simulink model "miniproject2"  (R2015a)
settings: Solver=ode45  StartTime=0.0  StopTime=0.1  RelTol=1e-3
undefined symbols (not defined in the file): D1, Delta
libraries: powerlib x18, powerlib_meascontrol x4
settings Model: Creator=ASUS  LastModifiedBy=ASUS

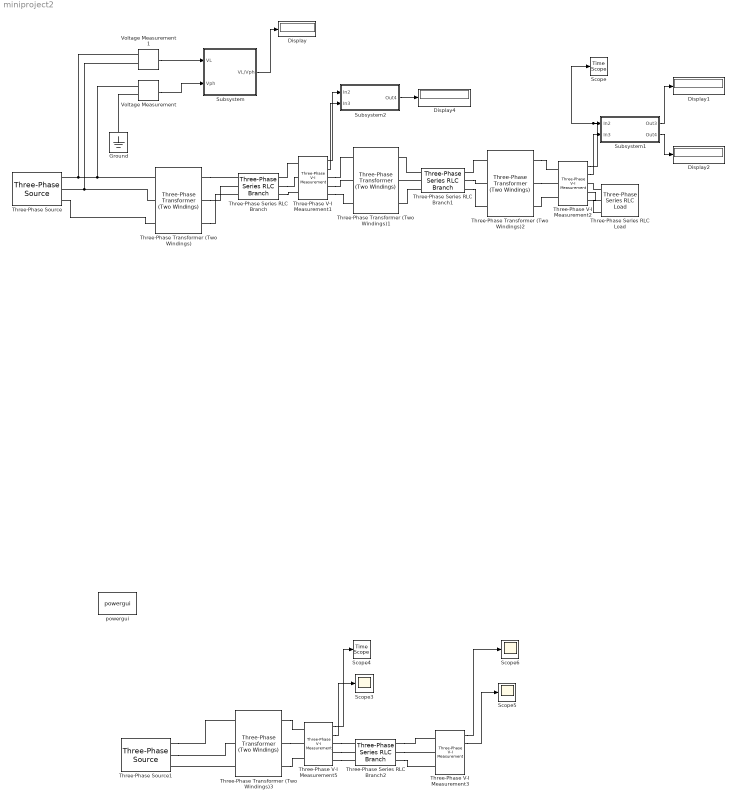
== system miniproject2 ==
  Display{,1..2,4} (4 alike) : Display
  Ground : powerlib/Elements/Ground  LConnTagsString=a
  Scope : TimeScope
  Scope3 : Scope
      settings: SaveName=ScopeData3
  Scope4 : TimeScope
  Scope5 : Scope
      settings: SaveName=ScopeData5
  Scope6 : Scope
      settings: SaveName=ScopeData8
  Subsystem : Subsystem
  Subsystem1 : Subsystem
  Subsystem2 : Subsystem
  Three-Phase Series RLC Branch : powerlib/Elements/Three-Phase Series RLC Branch  LConnTagsString=A|B|C  RConnTagsString=A|B|C  BranchType=RL  Resistance=271*0.01  Inductance=271*0.01  Capacitance=1e-6  Measurements=None
  Three-Phase Series RLC Branch1 : powerlib/Elements/Three-Phase Series RLC Branch  LConnTagsString=A|B|C  RConnTagsString=A|B|C  BranchType=RL  Resistance=(5+10^-3*171)  Inductance=(5+10^-3*171)  Capacitance=1e-6  Measurements=None
  Three-Phase Series RLC Branch2 : powerlib/Elements/Three-Phase Series RLC Branch  LConnTagsString=A|B|C  RConnTagsString=A|B|C  BranchType=RL  Resistance=271*0.01  Inductance=271*0.01  Capacitance=1e-6  Measurements=None
  Three-Phase Series RLC Load : powerlib/Elements/Three-Phase Series RLC Load  LConnTagsString=A|B|C  Configuration=Y (grounded)  NominalVoltage=1000  NominalFrequency=50  ActivePower=1000000  InductivePower=0.5e6  CapacitivePower=0  Measurements=None  LoadType=constant Z
  Three-Phase Transformer (Two Windings) : powerlib/Elements/Three-Phase Transformer (Two Windings)  Winding1Connection=Delta (D1)  Winding2Connection=Yg  CoreType=Three single-phase transformers  SetSaturation=off  Hysteresis=off  DataFile='hysteresis'  SetInitialFlux=off  Measurements=None  UNITS=pu  NominalPower=[ 250e6 , 50 ]  Winding1=[11000 0.0013774 17.309]  Winding2=[2.3e+05 9.4518e-06 0.11877]  Rm=344.35  Lm=1.0818e+05  L0=108.18  Saturation=[0 0;2.2401e-07 0.024234;9.3338e-05 0.030696]  InitialFluxes=[0.016156 -0.016156 0.014136]  MoreParameters=off  BreakLoop=off  DataType=off  TransfoNumber=1
  Three-Phase Transformer (Two Windings)1 : powerlib/Elements/Three-Phase Transformer (Two Windings)  Winding1Connection=Yg  Winding2Connection=Delta (D1)  CoreType=Three single-phase transformers  SetSaturation=off  Hysteresis=off  DataFile='hysteresis'  SetInitialFlux=off  Measurements=None  UNITS=SI  NominalPower=[ 450e6 , 50 ]  Winding1=[2.3e+05 6.5308e-07 5.8508e-13]  Winding2=[11000 2.2295e+09 1997.4]  Rm=0.16327  Lm=3.6568e-09  L0=8.2715e-07  Saturation=[0 0;6.901e+11 2523.6;2.8755e+14 3196.6]  InitialFluxes=[1682.4 -1682.4 1472.1]  MoreParameters=off  BreakLoop=off  DataType=on  TransfoNumber=1
  Three-Phase Transformer (Two Windings)2 : powerlib/Elements/Three-Phase Transformer (Two Windings)  Winding1Connection=Yg  Winding2Connection=Yg  CoreType=Three single-phase transformers  SetSaturation=off  Hysteresis=off  DataFile='hysteresis'  SetInitialFlux=off  Measurements=None  UNITS=pu  NominalPower=[ 450e6 , 50 ]  Winding1=[11000 0.007438 93.469]  Winding2=[400 5.625 70686]  Rm=1859.5  Lm=5.8418e+05  L0=584.18  Saturation=[0 0;7.1852e-08 0.041974;2.9938e-05 0.053168]  InitialFluxes=[0.027983 -0.027983 0.024485]  MoreParameters=off  BreakLoop=off  DataType=off  TransfoNumber=1
  Three-Phase Transformer (Two Windings)3 : powerlib/Elements/Three-Phase Transformer (Two Windings)  Winding1Connection=Delta (D1)  Winding2Connection=Yg  CoreType=Three single-phase transformers  SetSaturation=off  Hysteresis=off  DataFile='hysteresis'  SetInitialFlux=off  Measurements=None  UNITS=pu  NominalPower=[ 250e6 , 50 ]  Winding1=[11000 0.0013774 17.309]  Winding2=[2.3e+05 9.4518e-06 0.11877]  Rm=344.35  Lm=1.0818e+05  L0=108.18  Saturation=[0 0;2.2401e-07 0.024234;9.3338e-05 0.030696]  InitialFluxes=[0.016156 -0.016156 0.014136]  MoreParameters=off  BreakLoop=off  DataType=off  TransfoNumber=1
  Three-Phase V-I Measurement{1..3,5} (4 alike) : powerlib/Measurements/Three-Phase V-I Measurement  VoltageMeasurement=phase-to-ground  SetLabelV=off  LabelV=Vabc  Vpu=off  VpuLL=off  CurrentMeasurement=yes  SetLabelI=off  LabelI=Iabc  Ipu=off  Pbase=100e6  Vbase=500e3  OutputType=Complex  PhasorSimulation=off  PSBequivalent=0
  Three-Phase Source : powerlib/Electrical Sources/Three-Phase Source  Voltage=11000  PhaseAngle=0  Frequency=50  InternalConnection=Yg  SpecifyImpedance=off  Resistance=0  Inductance=0  ShortCircuitLevel=100e6  BaseVoltage=25e3  XRratio=7  BusType=swing  Pref=0  Qref=0  Qmin=-inf  Qmax=inf
  Three-Phase Source1 : powerlib/Electrical Sources/Three-Phase Source  Voltage=11000  PhaseAngle=0  Frequency=50  InternalConnection=Yg  SpecifyImpedance=off  Resistance=0  Inductance=0  ShortCircuitLevel=100e6  BaseVoltage=25e3  XRratio=7  BusType=swing  Pref=0  Qref=0  Qmin=-inf  Qmax=inf
  Voltage Measurement : powerlib/Measurements/Voltage Measurement  PhasorSimulation=off  OutputType=Complex  PSBequivalent=0
  Voltage Measurement1 : powerlib/Measurements/Voltage Measurement  PhasorSimulation=off  OutputType=Complex  PSBequivalent=0
  powergui : powerlib/powergui  Priority=1  SimulationMode=Continuous  SolverType=Tustin/Backward Euler (TBE)  SampleTime=50e-6  frequency=60  SPID=off  DisableSnubberDevices=off  DisableRonSwitches=off  DisableVfSwitches=off  SwTol=0  DisplayEquations=off  Interpol=off  methode=off  Ts=100  FunctionMessages=off  echomessages=off  HookPort=off  EnableUseOfTLC=off  x0status=blocks  frequencyindice=50  Pbase=100e6  ErrMax=1e-4  Iterations=50  UnitsV=kV  UnitsW=MW  buscounter=0  RestoreLinks=warning  ResistiveCurrentMeasurement=off  Frange=[0:2:500]  Ylog=off  Xlog=on  ShowGrid=off  save=off  variable=ZData  structure=0  ZoomFFT=off  StartTime=0.0  cycles=1  DisplayStyle=1  fundamental=60  FreqAxis=off  MaxFrequency=1000  frequencyindicesteady=1  RmsSteady=1  display=off
  wires:
  Voltage Measurement1/1 -> Subsystem/1(VL)
  Voltage Measurement/1 -> Subsystem/2(Vph)
  Subsystem/1(VL/Vph) -> Display/1
  Three-Phase V-I Measurement2/1 -> Scope/1, Subsystem1/1(In2)
  Three-Phase V-I Measurement2/2 -> Subsystem1/2(In3)
  Subsystem1/2(Out4) -> Display2/1
  Subsystem1/1(Out3) -> Display1/1
  Subsystem2/1(Out4) -> Display4/1
  Three-Phase V-I Measurement1/1 -> Subsystem2/1(In2)
  Three-Phase V-I Measurement1/2 -> Subsystem2/2(In3)
  Three-Phase V-I Measurement5/1 -> Scope4/1
  Three-Phase V-I Measurement5/2 -> Scope3/1
  Three-Phase V-I Measurement3/2 -> Scope5/1
  Three-Phase V-I Measurement3/1 -> Scope6/1
  connections:
  Three-Phase Transformer (Two Windings)/RConn2 -- Three-Phase Series RLC Branch/LConn2
  Three-Phase Series RLC Branch1/RConn2 -- Three-Phase Transformer (Two Windings)2/LConn2
  Three-Phase Transformer (Two Windings)/RConn3 -- Three-Phase Series RLC Branch/LConn3
  Three-Phase Transformer (Two Windings)2/RConn2 -- Three-Phase V-I Measurement2/LConn2
  Three-Phase Transformer (Two Windings)/LConn1 -- Three-Phase Source/RConn1 -- Voltage Measurement1/LConn1 -- Voltage Measurement/LConn1
  Three-Phase Transformer (Two Windings)/LConn2 -- Voltage Measurement1/LConn2 -- Three-Phase Source/RConn2
  Three-Phase Source/RConn3 -- Three-Phase Transformer (Two Windings)/LConn3
  Three-Phase Series RLC Branch1/LConn1 -- Three-Phase Transformer (Two Windings)1/RConn1
  Three-Phase Series RLC Load/LConn1 -- Three-Phase V-I Measurement2/RConn1
  Three-Phase Series RLC Branch1/RConn3 -- Three-Phase Transformer (Two Windings)2/LConn3
  Three-Phase V-I Measurement2/RConn3 -- Three-Phase Series RLC Load/LConn3
  Three-Phase Series RLC Branch1/LConn2 -- Three-Phase Transformer (Two Windings)1/RConn2
  Three-Phase Transformer (Two Windings)2/RConn3 -- Three-Phase V-I Measurement2/LConn3
  Three-Phase V-I Measurement2/RConn2 -- Three-Phase Series RLC Load/LConn2
  Three-Phase Series RLC Branch1/RConn1 -- Three-Phase Transformer (Two Windings)2/LConn1
  Three-Phase Transformer (Two Windings)1/RConn3 -- Three-Phase Series RLC Branch1/LConn3
  Ground/LConn1 -- Voltage Measurement/LConn2
  Three-Phase Transformer (Two Windings)/RConn1 -- Three-Phase Series RLC Branch/LConn1
  Three-Phase Transformer (Two Windings)2/RConn1 -- Three-Phase V-I Measurement2/LConn1
  Three-Phase Series RLC Branch/RConn1 -- Three-Phase V-I Measurement1/LConn1
  Three-Phase Series RLC Branch/RConn2 -- Three-Phase V-I Measurement1/LConn2
  Three-Phase Series RLC Branch/RConn3 -- Three-Phase V-I Measurement1/LConn3
  Three-Phase V-I Measurement1/RConn3 -- Three-Phase Transformer (Two Windings)1/LConn3
  Three-Phase V-I Measurement1/RConn2 -- Three-Phase Transformer (Two Windings)1/LConn2
  Three-Phase V-I Measurement1/RConn1 -- Three-Phase Transformer (Two Windings)1/LConn1
  Three-Phase Series RLC Branch2/RConn2 -- Three-Phase V-I Measurement3/LConn2
  Three-Phase Series RLC Branch2/RConn3 -- Three-Phase V-I Measurement3/LConn3
  Three-Phase Series RLC Branch2/RConn1 -- Three-Phase V-I Measurement3/LConn1
  Three-Phase Source1/RConn2 -- Three-Phase Transformer (Two Windings)3/LConn2
  Three-Phase Source1/RConn1 -- Three-Phase Transformer (Two Windings)3/LConn1
  Three-Phase Transformer (Two Windings)3/LConn3 -- Three-Phase Source1/RConn3
  Three-Phase Transformer (Two Windings)3/RConn1 -- Three-Phase V-I Measurement5/LConn1
  Three-Phase Transformer (Two Windings)3/RConn2 -- Three-Phase V-I Measurement5/LConn2
  Three-Phase Transformer (Two Windings)3/RConn3 -- Three-Phase V-I Measurement5/LConn3
  Three-Phase V-I Measurement5/RConn1 -- Three-Phase Series RLC Branch2/LConn1
  Three-Phase V-I Measurement5/RConn2 -- Three-Phase Series RLC Branch2/LConn2
  Three-Phase V-I Measurement5/RConn3 -- Three-Phase Series RLC Branch2/LConn3

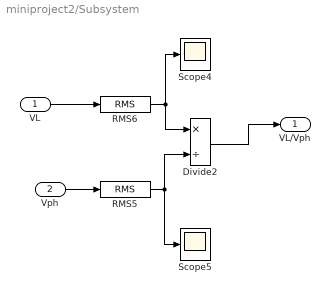
== system miniproject2/Subsystem ==
  VL : Inport
  Vph : Inport  Port=2
  Divide2 : Product  Inputs=*/
  RMS5 : powerlib_meascontrol/Measurements/RMS  TrueRMS=on  Freq=50  RMSInit=0  Ts=0
  RMS6 : powerlib_meascontrol/Measurements/RMS  TrueRMS=on  Freq=50  RMSInit=0  Ts=0
  Scope4 : Scope
      settings: SaveName=ScopeData6
  Scope5 : Scope
      settings: SaveName=ScopeData7
  VL/Vph : Outport
  wires:
  RMS6/1 -> Scope4/1, Divide2/1
  RMS5/1 -> Scope5/1, Divide2/2
  Divide2/1 -> VL/Vph/1
  VL/1 -> RMS6/1
  Vph/1 -> RMS5/1

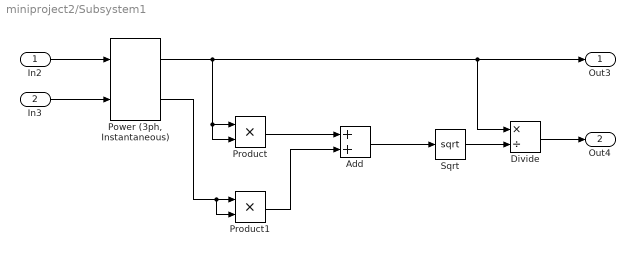
== system miniproject2/Subsystem1 ==
  In2 : Inport
  In3 : Inport  Port=2
  Add : Sum
  Divide : Product  Inputs=*/
  "Power (3ph, Instantaneous)" : powerlib_meascontrol/Measurements/Power (3ph, Instantaneous)
  Product : Product
  Product1 : Product
  Sqrt : Sqrt  SaturateOnIntegerOverflow=on
  Out3 : Outport
  Out4 : Outport  Port=2
  wires:
  In3/1 -> "Power (3ph, Instantaneous)"/2
  "Power (3ph, Instantaneous)"/2 -> Product1/2, Product1/1
  Product1/1 -> Add/2
  Add/1 -> Sqrt/1
  Product/1 -> Add/1
  Sqrt/1 -> Divide/2
  In2/1 -> "Power (3ph, Instantaneous)"/1
  Divide/1 -> Out4/1
  "Power (3ph, Instantaneous)"/1 -> Product/2, Product/1, Divide/1, Out3/1

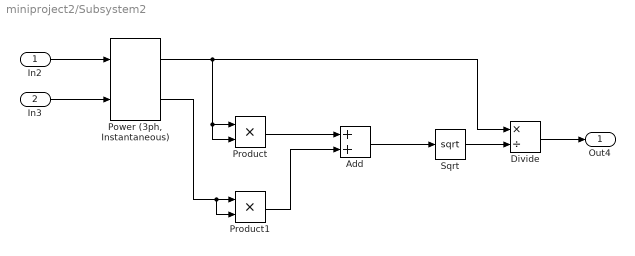
== system miniproject2/Subsystem2 ==
  In2 : Inport
  In3 : Inport  Port=2
  Add : Sum
  Divide : Product  Inputs=*/
  "Power (3ph, Instantaneous)" : powerlib_meascontrol/Measurements/Power (3ph, Instantaneous)
  Product : Product
  Product1 : Product
  Sqrt : Sqrt  SaturateOnIntegerOverflow=on
  Out4 : Outport
  wires:
  In3/1 -> "Power (3ph, Instantaneous)"/2
  "Power (3ph, Instantaneous)"/2 -> Product1/2, Product1/1
  Product1/1 -> Add/2
  Add/1 -> Sqrt/1
  Product/1 -> Add/1
  Sqrt/1 -> Divide/2
  In2/1 -> "Power (3ph, Instantaneous)"/1
  Divide/1 -> Out4/1
  "Power (3ph, Instantaneous)"/1 -> Product/2, Product/1, Divide/1
